simulink model "model"  (R2021a)
settings: Solver=VariableStepAuto  StartTime=0.0  StopTime=20.0  RelTol=1e-3
libraries: robotmobilelib x1, simulink x1
settings Model: Creator=admin  LastModifiedBy=admin

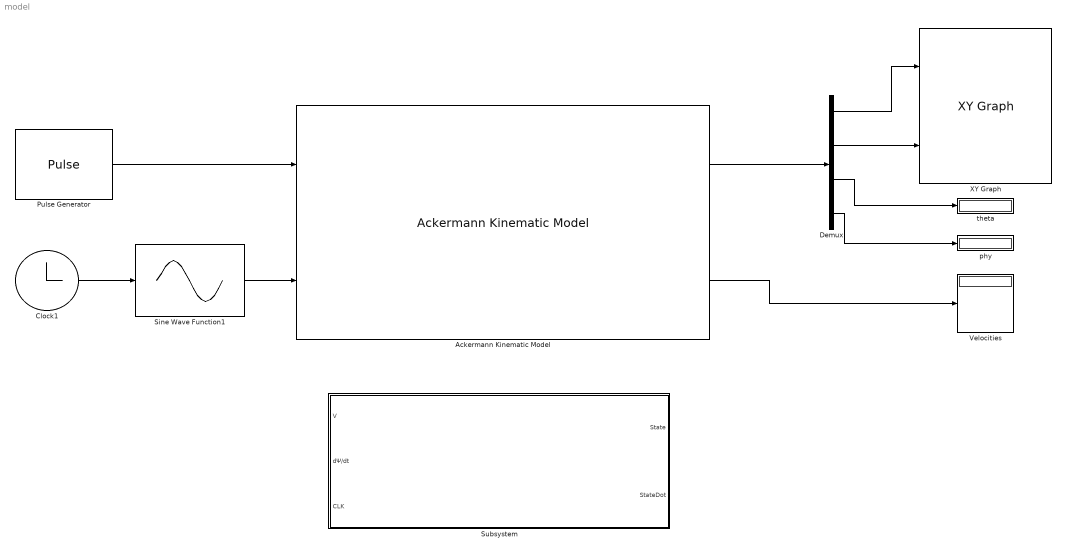
== system model ==
  Ackermann Kinematic Model : robotmobilelib/Ackermann Kinematic Model  WheelBase=2.2  VehicleSpeedRange=[-5.556 -5.556]  MaxSteeringAngle=pi/4  InitialState=[0; 0; 0; 0]  SimulateUsing=Interpreted execution
      settings: SourceProductBaseCode=RO
  Clock1 : Clock
  Demux : Demux
  Pulse Generator : DiscretePulseGenerator  PulseType=Time based  Period=5  PulseWidth=5
  Sine Wave Function1 : Sin  TimeSource=Use external signal  Amplitude=pi/12  Frequency=2*pi/5  SampleTime=0
  Subsystem : Subsystem
  Velocities : Display
  XY Graph : simulink/Sinks/XY Graph  xmin=-30  xmax=30  ymin=-30  ymax=30  st=0.001
  phy : Display
  theta : Display
  wires:
  Ackermann Kinematic Model/1 -> Demux/1
  Demux/2 -> XY Graph/2
  Demux/1 -> XY Graph/1
  Demux/3 -> theta/1
  Demux/4 -> phy/1
  Ackermann Kinematic Model/2 -> Velocities/1
  Pulse Generator/1 -> Ackermann Kinematic Model/1
  Clock1/1 -> Sine Wave Function1/1
  Sine Wave Function1/1 -> Ackermann Kinematic Model/2

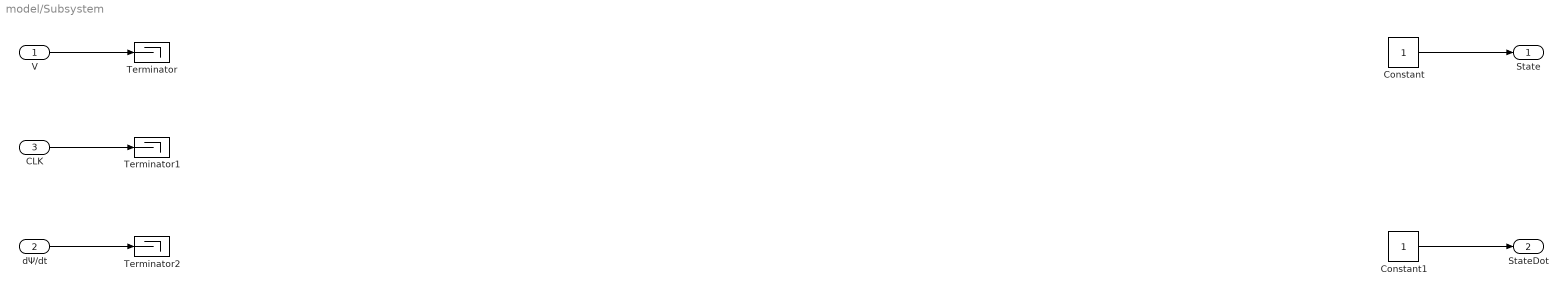
== system model/Subsystem ==
  V : Inport
  dΨ/dt : Inport  Port=2
  CLK : Inport  Port=3
  Constant : Constant
  Constant1 : Constant
  Terminator : Terminator
  Terminator1 : Terminator
  Terminator2 : Terminator
  State : Outport
  StateDot : Outport  Port=2
  wires:
  V/1 -> Terminator/1
  dΨ/dt/1 -> Terminator2/1
  CLK/1 -> Terminator1/1
  Constant/1 -> State/1
  Constant1/1 -> StateDot/1
